simulink model "Wiper_system"  (R2022b)
settings: Solver=FixedStepDiscrete  StartTime=0.0  StopTime=50  FixedStep=1e-3  RelTol=1e-3
undefined symbols (not defined in the file or in its folder): sigbuilder_block
libraries: pil_lib x1
settings Model: Creator=Dell  LastModifiedBy=Dell
settings DataIOCC: SaveFormat=Array  OutputSaveName=SIL_out  LoggingToFile=on  LoggingFileName=SIL_out.mat
settings OptimizationCC: DefaultParameterBehavior=Inlined  UseDivisionForNetSlopeComputation=on  GainParamInheritBuiltInType=on  UseFloatMulNetSlope=on  InlineInvariantSignals=on  PassReuseOutputArgsAs=Individual arguments  ZeroExternalMemoryAtStartup=off  ZeroInternalMemoryAtStartup=off  NoFixptDivByZeroProtection=on  EfficientFloat2IntCast=on  LifeSpan=1  OptimizeBlockOrder=speed  DifferentSizesBufferReuse=on  EfficientTunableParamExpr=on
settings DebuggingCC: ParameterTunabilityLossMsg=error
settings HardwareCC: ProdBitPerPointer=32  ProdBitPerSizeT=32  ProdBitPerPtrDiffT=32  ProdLargestAtomicInteger=Long  ProdLargestAtomicFloat=Double  ProdWordSize=32  ProdLongLongMode=on  ProdHWDeviceType=ARM Compatible->ARM Cortex-M
settings SFSimCC: MATLABDynamicMemAlloc=off
settings RTWCC: Description=Embedded Coder  SystemTargetFile=ert.tlc  TemplateMakefile=ert_default_tmf
settings CodeAppCC: ForceParamTrailComments=on  IgnoreCustomStorageClasses=off  OperatorAnnotations=on  SimulinkDataObjDesc=on  SFDataObjDesc=on  CustomSymbolStrGlobalVar=rt$N$M  CustomSymbolStrType=$N$M  CustomSymbolStrFcn=$N$M$F  CustomSymbolStrMacro=$N$M  InsertBlockDesc=on
settings ERTTargetCC: TargetLangStandard=C99 (ISO)  GenerateSampleERTMain=on  IncludeMdlTerminateFcn=off  CombineSignalStateStructs=on  SupportComplex=off  SupportContinuousTime=on  InlinedParameterPlacement=NonHierarchical  ERTCustomFileTemplate=example_file_process.tlc  ERTFilePackagingFormat=CompactWithDataFile

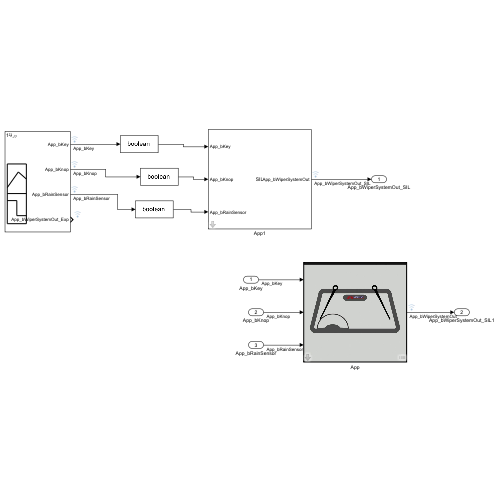
[thumbnail: Simulink's stored preview of the top-level diagram]
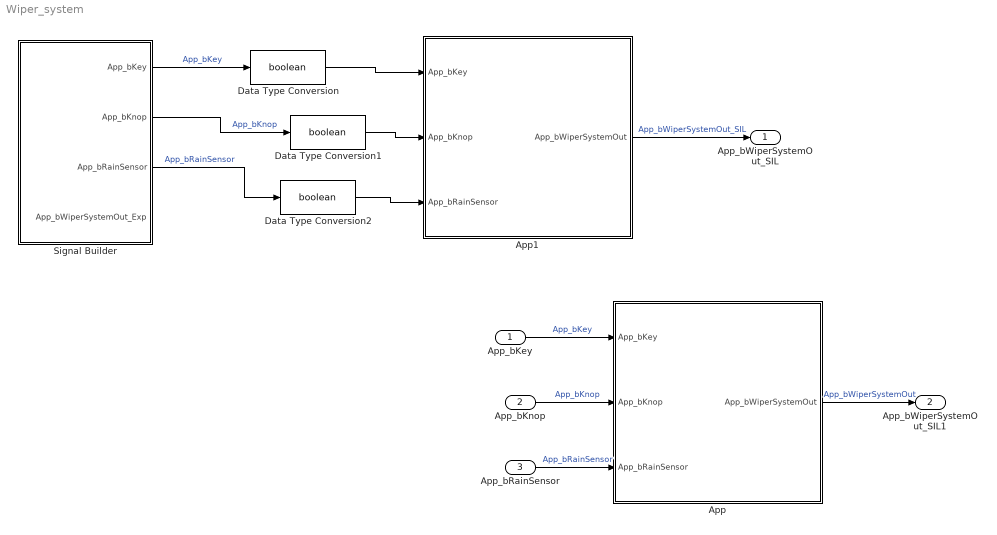
== system Wiper_system ==
  App_bKey : Inport
  App_bKnop : Inport  Port=2
  App_bRainSensor : Inport  Port=3
  App : Subsystem  TreatAsAtomicUnit=on
      mask Display: image('wiper.jpg');
  App1 : Subsystem  Tag=__SL_testing_harness_stub_  DialogController=pil_create_dialog  LoadFcn=|
      | try
      |    if ~strcmp(rtw.pil.getPILVersion, '9.13 (R2022b)_15')
      |       set_param(gcb, 'DialogController', '');
      |       set_param(gcb, 'DialogControllerArgs', '');
      |    end
      | catch e
      |       set_param(gcb, 'DialogController', '');
      |       set_param(gcb, 'DialogControllerArgs', '');
      | end
      mask help: PIL:pil:XILBlockMaskDesc
      mask Display: disp('SIL');
  Data Type Conversion : DataTypeConversion  OutDataTypeStr=boolean  SaturateOnIntegerOverflow=off  RndMeth=Floor
  Data Type Conversion1 : DataTypeConversion  OutDataTypeStr=boolean  SaturateOnIntegerOverflow=off  RndMeth=Floor
  Data Type Conversion2 : DataTypeConversion  OutDataTypeStr=boolean  SaturateOnIntegerOverflow=off  RndMeth=Floor
  Signal Builder : Subsystem  Tag=STV Subsys  LoadFcn=sigbuilder_block('load');  StartFcn=sigbuilder_block('start');  StopFcn=sigbuilder_block('stop');  ClipboardFcn=sigbuilder_block('clipboard');  mask(Sigbuilder block){tuvar=[0:10]}
      mask help: Simulink:masks:SigbuilderBlock_MD
      mask init:
      | if ~strcmp(get_param(bdroot(gcbh),'SimulationStatus'),'stopped') tuvar = sigbuilder_block('maskInit'); end
      settings: CopyFcn=sigbuilder_block('copy');  DeleteFcn=sigbuilder_block('delete');  ModelCloseFcn=sigbuilder_block('modelClose');  PreSaveFcn=sigbuilder_block('preSave');  PauseFcn=sigbuilder_block('pause');  ContinueFcn=sigbuilder_block('continue');  NameChangeFcn=sigbuilder_block('namechange');  OpenFcn=sigbuilder_block('open',[437.6 199.2 550.4 400 ]);  CloseFcn=sigbuilder_block('close');
      mask Display: plot(0, 0, 100, 100,[2, 2, 32, 32, 2], [68, 8, 8, 68, 68],[32, 2], [38, 38], [32, 19, 2],[53, 60, 44], [32, 17, 17, 2],[16, 16, 31, 31]);txt = getActiveGroup(gcbh);text(2, 100, txt,'verticalAlignment', 'top');
  App_bWiperSystemOut_SIL : Outport
  App_bWiperSystemOut_SIL1 : Outport  Port=2
  wires:
  Signal Builder/1(App_bKey) -> Data Type Conversion/1  "App_bKey"
  Signal Builder/2(App_bKnop) -> Data Type Conversion1/1  "App_bKnop"
  Signal Builder/3(App_bRainSensor) -> Data Type Conversion2/1  "App_bRainSensor"
  Data Type Conversion/1 -> App1/1(App_bKey)
  Data Type Conversion1/1 -> App1/2(App_bKnop)
  Data Type Conversion2/1 -> App1/3(App_bRainSensor)
  App1/1(App_bWiperSystemOut) -> App_bWiperSystemOut_SIL/1  "App_bWiperSystemOut_SIL"
  App_bKey/1 -> App/1(App_bKey)  "App_bKey"
  App_bKnop/1 -> App/2(App_bKnop)  "App_bKnop"
  App_bRainSensor/1 -> App/3(App_bRainSensor)  "App_bRainSensor"
  App/1(App_bWiperSystemOut) -> App_bWiperSystemOut_SIL1/1  "App_bWiperSystemOut"

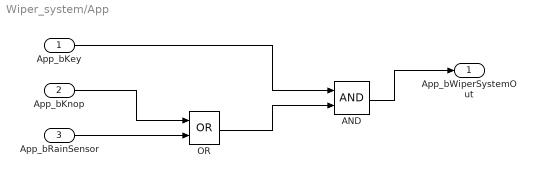
== system Wiper_system/App ==
  App_bKey : Inport
  App_bKnop : Inport  Port=2
  App_bRainSensor : Inport  Port=3
  AND : Logic  AllPortsSameDT=off  OutDataTypeStr=boolean
  OR : Logic  Operator=OR  AllPortsSameDT=off  OutDataTypeStr=boolean
  App_bWiperSystemOut : Outport
  wires:
  App_bKnop/1 -> OR/1
  App_bRainSensor/1 -> OR/2
  App_bKey/1 -> AND/1
  OR/1 -> AND/2
  AND/1 -> App_bWiperSystemOut/1

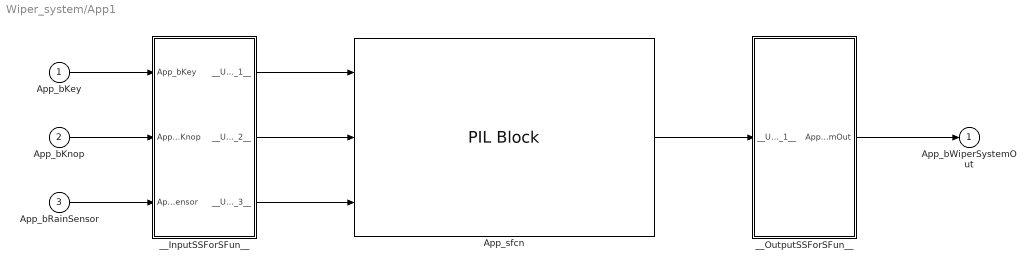
== system Wiper_system/App1 ==
  App_bKey : Inport
  App_bKnop : Inport  Port=2
  App_bRainSensor : Inport  Port=3
  App_sfcn : pil_lib/PIL Block  SimulationMode=SIL  IsTopModelPIL=off  CodeDir=App_ert_rtw  AnchorDir=E:\MBD  ConfigName=Software-in-the-Loop (SIL)  XrelIsTopModelCode=on  XrelIsReusable=off  XrelDWorkNames={}  XrelDWorkTypes={}  XrelModelArgVals={}  XrelOrderedParamNames={}
  __InputSSForSFun__ : Subsystem
  __OutputSSForSFun__ : Subsystem
  App_bWiperSystemOut : Outport
  wires:
  __OutputSSForSFun__/1(App_bWiperSystemOut) -> App_bWiperSystemOut/1
  App_sfcn/1 -> __OutputSSForSFun__/1(__UniqueInportName__1__)
  __InputSSForSFun__/3(__UniqueOutportName__3__) -> App_sfcn/3
  __InputSSForSFun__/2(__UniqueOutportName__2__) -> App_sfcn/2
  __InputSSForSFun__/1(__UniqueOutportName__1__) -> App_sfcn/1
  App_bRainSensor/1 -> __InputSSForSFun__/3(App_bRainSensor)
  App_bKnop/1 -> __InputSSForSFun__/2(App_bKnop)
  App_bKey/1 -> __InputSSForSFun__/1(App_bKey)

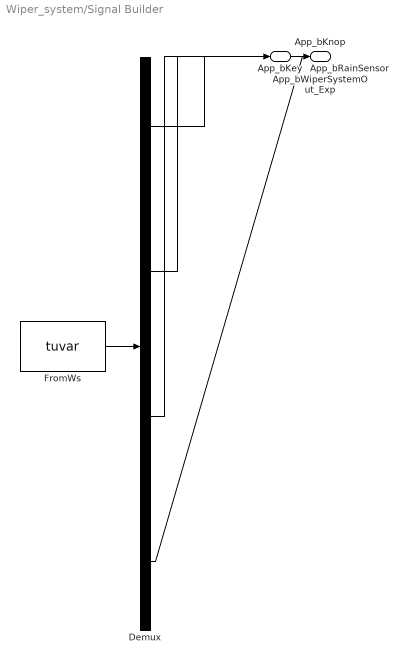
== system Wiper_system/Signal Builder ==
  Demux : Demux  Tag=STV Demux
      settings: DisplayOption=none
  FromWs : FromWorkspace  Tag=STV FromWs  VariableName=tuvar
      SigBuilderData=|
      | common.afterFinalStr = 'Extrapolate'
      | common.sampleTime = 0
      | dataSet.timeRange = [0 45]
      | dataSet.name = 'ورقة1'
      | sbobj.Name = 'Signal Builder'
      | sbobj.Groups.Name = 'ورقة1'
      | sbobj.Groups.Signals(1).Name = 'App_bKey'
      | sbobj.Groups.Signals(1).XData = [0 5 5 10 10 20 20 30 30 35 35 40 40 45]
      | sbobj.Groups.Signals(1).YData = [0 0 1 1 1 1 1 1 0 0 0 0 1 1]
      | sbobj.Groups.Signals(2).Name = 'App_bKnop'
      | sbobj.Groups.Signals(2).XData = [0 5 10 10 20 20 30 35 35 40 45]
      | sbobj.Groups.Signals(2).YData = [0 0 0 1 1 0 0 0 1 1 1]
      | sbobj.Groups.Signals(3).Name = 'App_bRainSensor'
      | sbobj.Groups.Signals(3).XData = [0 5 10 20 20 30 35 40 45]
      | sbobj.Groups.Signals(3).YData = [0 0 0 0 1 1 1 1 1]
      | sbobj.Groups.Signals(4).Name = 'App_bWiperSystemOut_Exp'
      | sbobj.Groups.Signals(4).XData = [0 5 10 10 20 30 30 35 40 40 45]
      | sbobj.Groups.Signals(4).YData = [0 0 0 1 1 1 0 0 0 1 1]
      | sbobj.Groups.TimeRange = [0 45]
  App_bKey : Outport  Tag=STV Outport
  App_bKnop : Outport  Tag=STV Outport  Port=2
  App_bRainSensor : Outport  Tag=STV Outport  Port=3
  App_bWiperSystemOut_Exp : Outport  Tag=STV Outport  Port=4
  wires:
  Demux/1 -> App_bKey/1
  FromWs/1 -> Demux/1
  Demux/2 -> App_bKnop/1
  Demux/3 -> App_bRainSensor/1
  Demux/4 -> App_bWiperSystemOut_Exp/1

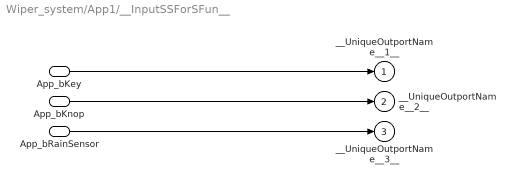
== system Wiper_system/App1/__InputSSForSFun__ ==
  App_bKey : Inport
  App_bKnop : Inport  Port=2
  App_bRainSensor : Inport  Port=3
  __UniqueOutportName__1__ : Outport
  __UniqueOutportName__2__ : Outport  Port=2
  __UniqueOutportName__3__ : Outport  Port=3
  wires:
  App_bRainSensor/1 -> __UniqueOutportName__3__/1
  App_bKnop/1 -> __UniqueOutportName__2__/1
  App_bKey/1 -> __UniqueOutportName__1__/1

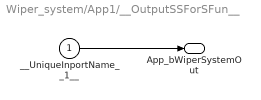
== system Wiper_system/App1/__OutputSSForSFun__ ==
  __UniqueInportName__1__ : Inport
  App_bWiperSystemOut : Outport
  wires:
  __UniqueInportName__1__/1 -> App_bWiperSystemOut/1
